simulink model "Zadatak2"  (R2023a)
settings: Solver=VariableStepAuto  StartTime=0.0  StopTime=T_sim  RelTol=1e-3
values from neighbouring files (symbols this model uses):
  K = 20    [Zadatak2_skripta.m]    (also in Zadatak2_skripta2.m)
  KR = n*pi/2 * T1/(T*K)    (= 0.113686384152)    [Zadatak2_skripta.m]    (also in Zadatak2_skripta2.m = 0.0942477796077)
  T = 2    [Zadatak2_skripta.m]    (also in Zadatak2_skripta2.m)
  T1 = 3    [Zadatak2_skripta.m]    (also in Zadatak2_skripta2.m)
  TR = T1    (= 3)    [Zadatak2_skripta.m]    (also in Zadatak2_skripta2.m)
  y_ref = 8    [Zadatak2_skripta.m]    (also in Zadatak2_skripta2.m = 11)
settings Model: Creator=Jure  LastModifiedBy=Enio
settings SolverCC: AlgebraicLoopSolver=TrustRegion
settings DataIOCC: ReturnWorkspaceOutputs=off
settings DebuggingCC: UnconnectedInputMsg=warning  UnconnectedOutputMsg=warning  UnconnectedLineMsg=warning  ArithmeticOperatorsInVariantConditions=warning
settings ModelReferenceCC: EnableRefExpFcnMdlSchedulingChecks=on
settings SFSimCC: CustomCodeUndefinedFunction=UseInterfaceOnly
settings RTWCC: DLArmComputeVersion=19.05

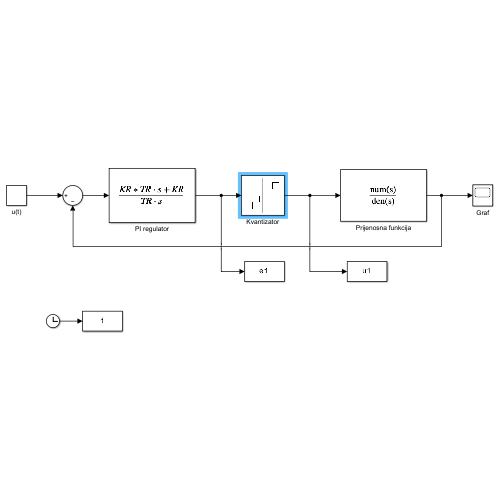
[thumbnail: Simulink's stored preview of the top-level diagram]
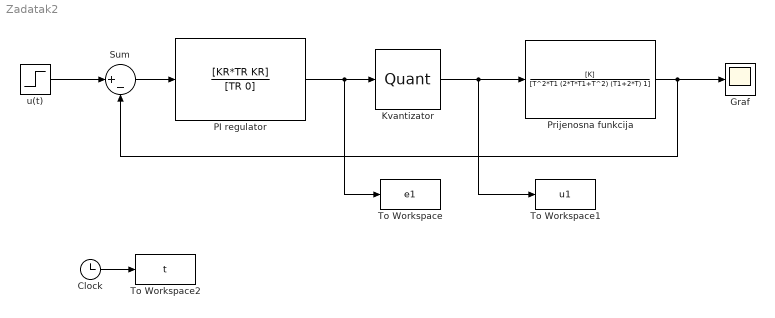
== system Zadatak2 ==
  Clock : Clock
  Graf : Scope
  Kvantizator : Quantizer  QuantizationInterval=D
  PI regulator : TransferFcn  Numerator=[KR*TR KR]  Denominator=[TR 0]
  Prijenosna funkcija : TransferFcn  Numerator=[K]  Denominator=[T^2*T1 (2*T*T1+T^2) (T1+2*T) 1]
  Sum : Sum  Inputs=|+-
  To Workspace : ToWorkspace  VariableName=e1  SampleTime=0.001
  To Workspace1 : ToWorkspace  VariableName=u1  SampleTime=0.001
  To Workspace2 : ToWorkspace  VariableName=t  SampleTime=0.001
  u(t) : Step  Time=0  After=y_ref  SampleTime=0
  wires:
  u(t)/1 -> Sum/1
  Sum/1 -> PI regulator/1
  PI regulator/1 -> Kvantizator/1, To Workspace/1
  Kvantizator/1 -> To Workspace1/1, Prijenosna funkcija/1
  Prijenosna funkcija/1 -> Sum/2, Graf/1
  Clock/1 -> To Workspace2/1
